simulink model "q1_b2"  (R2022a)
settings: Solver=VariableStepAuto  StartTime=0.0  StopTime=100  RelTol=1e-3
settings Model: Creator=Fujitsu  LastModifiedBy=ZahraIranpour
settings SolverCC: AlgebraicLoopSolver=TrustRegion
settings DataIOCC: ReturnWorkspaceOutputs=off
settings DebuggingCC: UnconnectedInputMsg=warning  UnconnectedOutputMsg=warning  UnconnectedLineMsg=warning  SFMachineParentedDataDiag=warning  ArithmeticOperatorsInVariantConditions=warning
settings SFSimCC: CustomCodeUndefinedFunction=UseInterfaceOnly

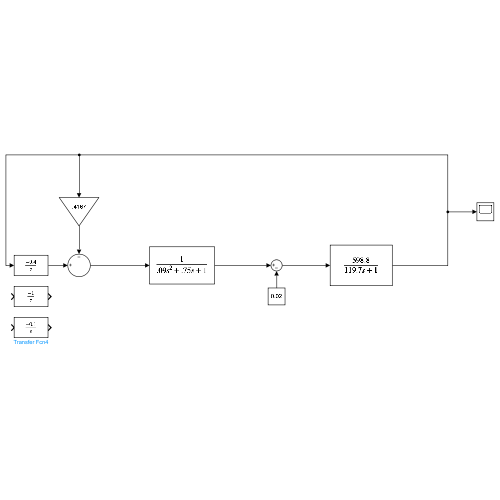
[thumbnail: Simulink's stored preview of the top-level diagram]
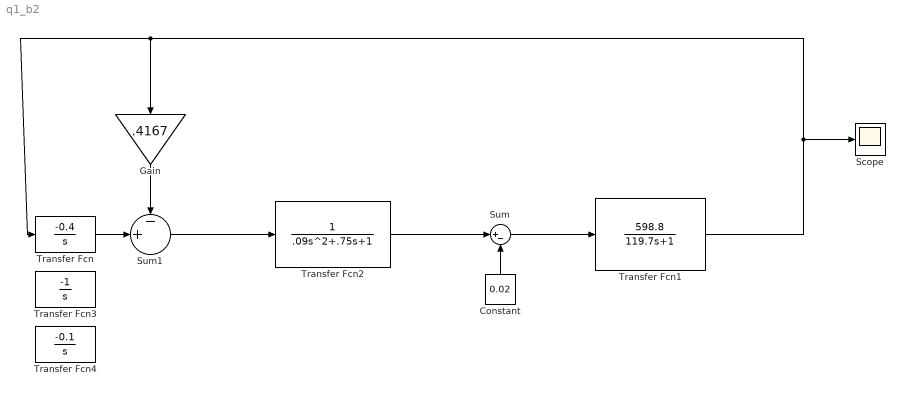
== system q1_b2 ==
  Constant : Constant  Value=0.02
  Gain : Gain  Gain=.4167
  Scope : Scope
  Sum : Sum  Inputs=|+-
  Sum1 : Sum  Inputs=-+|
  Transfer Fcn : TransferFcn  Numerator=[-0.4]  Denominator=[1 0]
  Transfer Fcn1 : TransferFcn  Numerator=[598.8]  Denominator=[119.7 1]
  Transfer Fcn2 : TransferFcn  Denominator=[.09 .75 1]
  Transfer Fcn3 : TransferFcn  Numerator=[-1]  Denominator=[1 0]
  Transfer Fcn4 : TransferFcn  Numerator=[-0.1]  Denominator=[1 0]
  wires:
  Transfer Fcn1/1 -> Scope/1, Transfer Fcn/1, Gain/1
  Sum1/1 -> Transfer Fcn2/1
  Transfer Fcn2/1 -> Sum/1
  Transfer Fcn/1 -> Sum1/2
  Constant/1 -> Sum/2
  Gain/1 -> Sum1/1
  Sum/1 -> Transfer Fcn1/1
